simulink model "VVI_Ready_For_Requirements"  (R2022a)
settings: Solver=FixedStepAuto  StartTime=0.0  StopTime=10.0  FixedStep=1e-3  RelTol=1e-3  EnableMultiTasking=on
undefined symbols (not defined in the file): D1, D10, D11, D12, D13, D2, D3, D4, D5, D7, D8, D9, PTA0, PTA1, PTA2, PTB23, PTB9, PTC17, PTC3, PTC4, PTD0, PTD1, PTD2, PTD3
libraries: frdmk64flib x12
settings Model: ExtModeTrigDuration=5  Creator=ethan  LastModifiedBy=ethan
settings OptimizationCC: EnhancedBackFolding=on  PassReuseOutputArgsAs=Individual arguments  ZeroExternalMemoryAtStartup=off  ZeroInternalMemoryAtStartup=off  MaxStackSize=64  OptimizeBlockOrder=speed  DifferentSizesBufferReuse=on  OptimizationCustomize=off  EfficientTunableParamExpr=on
settings DebuggingCC: ParameterTunabilityLossMsg=error
settings HardwareCC: ProdBitPerPointer=32  ProdBitPerSizeT=32  ProdBitPerPtrDiffT=32  ProdLargestAtomicInteger=Long  ProdLargestAtomicFloat=Double  ProdWordSize=32  ProdHWDeviceType=ARM Compatible->ARM Cortex
settings SFSimCC: MATLABDynamicMemAlloc=off
settings RTWCC: SystemTargetFile=ert.tlc  HardwareBoard=NXP FRDM-K64F  TLCOptions="-aInlineSetEventsForThisBaseRateFcn=TLC_FALSE -aSuppressMultiTaskScheduler=TLC_FALSE  -aRateBasedStepFcn=0"  TemplateMakefile=ert_default_tmf  Toolchain=GNU Tools for ARM Embedded Processors
settings CodeAppCC: ForceParamTrailComments=on  IgnoreCustomStorageClasses=off  OperatorAnnotations=on  SimulinkDataObjDesc=on  SFDataObjDesc=on  InsertBlockDesc=on
settings ERTTargetCC: ExtModeTransport=4  ExtModeMexFile=sendToCommService

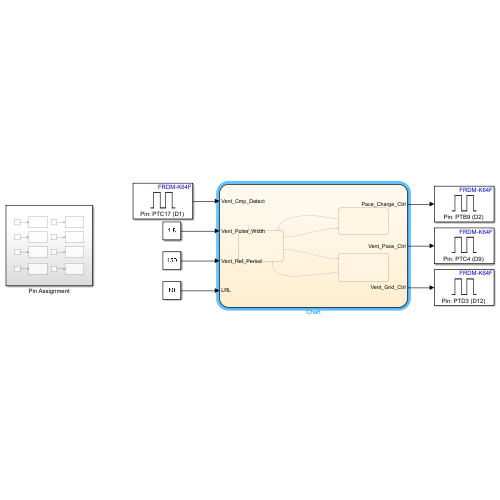
[thumbnail: Simulink's stored preview of the top-level diagram]
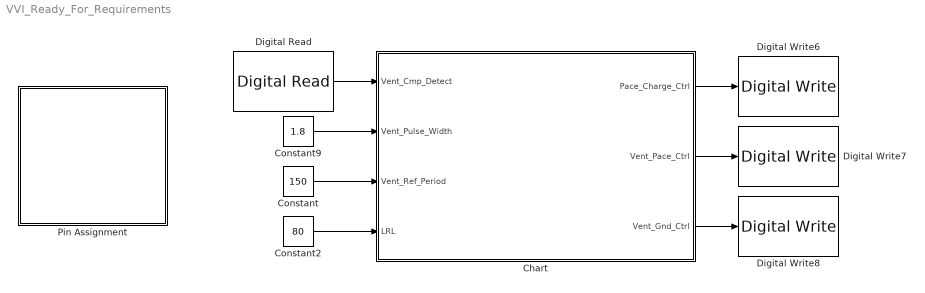
== system VVI_Ready_For_Requirements ==
  Chart : Stateflow chart  TreatAsAtomicUnit=on
  Constant : Constant  Value=150  OutDataTypeStr=int16
  Constant2 : Constant  Value=80
  Constant9 : Constant  Value=1.8
  Digital Read : frdmk64flib/Digital Read  Whichpin=PTC17 (D1)  SampleTime=-1
  Digital Write6 : frdmk64flib/Digital Write  Whichpin=PTB9 (D2)
  Digital Write7 : frdmk64flib/Digital Write  Whichpin=PTC4 (D9)
  Digital Write8 : frdmk64flib/Digital Write  Whichpin=PTD3 (D12)
  Pin Assignment : Subsystem
  wires:
  Chart/3(Vent_Gnd_Ctrl) -> Digital Write8/1
  Chart/2(Vent_Pace_Ctrl) -> Digital Write7/1
  Constant2/1 -> Chart/4(LRL)
  Constant9/1 -> Chart/2(Vent_Pulse_Width)
  Chart/1(Pace_Charge_Ctrl) -> Digital Write6/1
  Digital Read/1 -> Chart/1(Vent_Cmp_Detect)
  Constant/1 -> Chart/3(Vent_Ref_Period)

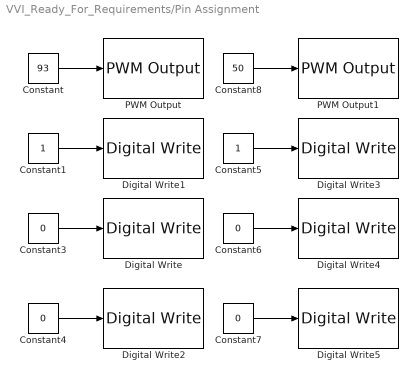
== system VVI_Ready_For_Requirements/Pin Assignment ==
  Constant : Constant  Value=93  OutDataTypeStr=int8
  Constant1 : Constant
  Constant{3..4,6..7} (4 alike) : Constant  Value=0
  Constant5 : Constant
  Constant8 : Constant  Value=50  OutDataTypeStr=int8
  Digital Write : frdmk64flib/Digital Write  Whichpin=PTB23 (D4)
  Digital Write1 : frdmk64flib/Digital Write  Whichpin=PTD1 (D13)
  Digital Write2 : frdmk64flib/Digital Write  Whichpin=PTC3 (D7)
  Digital Write3 : frdmk64flib/Digital Write  Whichpin=PTD0 (D10)
  Digital Write4 : frdmk64flib/Digital Write  Whichpin=PTD2 (D11)
  Digital Write5 : frdmk64flib/Digital Write  Whichpin=PTA0 (D8)
  PWM Output : frdmk64flib/PWM Output  Whichpin=PTA1 (D3)  InitialFrequency=2000  InitialDutyCycle=0
  PWM Output1 : frdmk64flib/PWM Output  Whichpin=PTA2 (D5)  InitialFrequency=2000  InitialDutyCycle=0
  wires:
  Constant1/1 -> Digital Write1/1
  Constant5/1 -> Digital Write3/1
  Constant7/1 -> Digital Write5/1
  Constant4/1 -> Digital Write2/1
  Constant/1 -> PWM Output/1
  Constant8/1 -> PWM Output1/1
  Constant3/1 -> Digital Write/1
  Constant6/1 -> Digital Write4/1

== stateflow chart VVI_Ready_For_Requirements/Chart ==
  state Inhibit
    entry:
    Vent_Pace_Ctrl = false;
    Vent_Gnd_Ctrl = true;
    Pace_Charge_Ctrl = true;
  state Signal_Search
    entry:
    Vent_Pace_Ctrl = false;
    Vent_Gnd_Ctrl = true;
    Pace_Charge_Ctrl = true;
  state Pace
    entry:
    Pace_Charge_Ctrl = false;
    Vent_Pace_Ctrl = true;
    Vent_Gnd_Ctrl = false;
  Inhibit -> Signal_Search : after(Vent_Ref_Period,msec)
  (default) -> Signal_Search
  Signal_Search -> Inhibit [order 2] : [Vent_Cmp_Detect == true]
  Signal_Search -> Pace [order 1] : [after(((60000/LRL)-Vent_Pulse_Width),msec)]
  Pace -> Signal_Search : after(Vent_Pulse_Width,msec)
  data: Vent_Cmp_Detect input boolean; Vent_Pulse_Width input; Vent_Ref_Period input; Pace_Charge_Ctrl output; Vent_Pace_Ctrl output; Vent_Gnd_Ctrl output; LRL input
